simulink model "sampleModel1530"  (R2023a)
settings: Solver=VariableStepAuto  StartTime=0.0  StopTime=10.0  RelTol=1e-3
libraries: hdlsllib x6, simulink x1
settings Model: Creator=user1  LastModifiedBy=user1

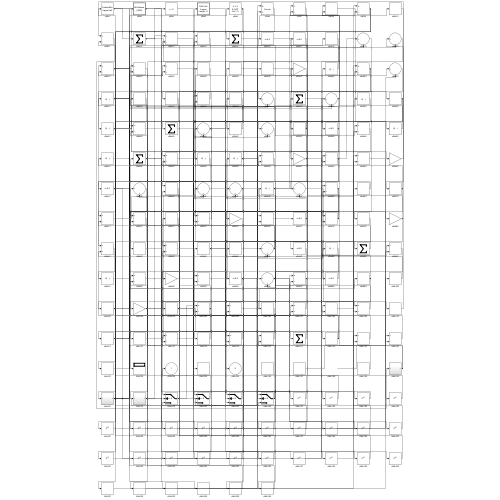
[thumbnail: Simulink's stored preview of the top-level diagram]
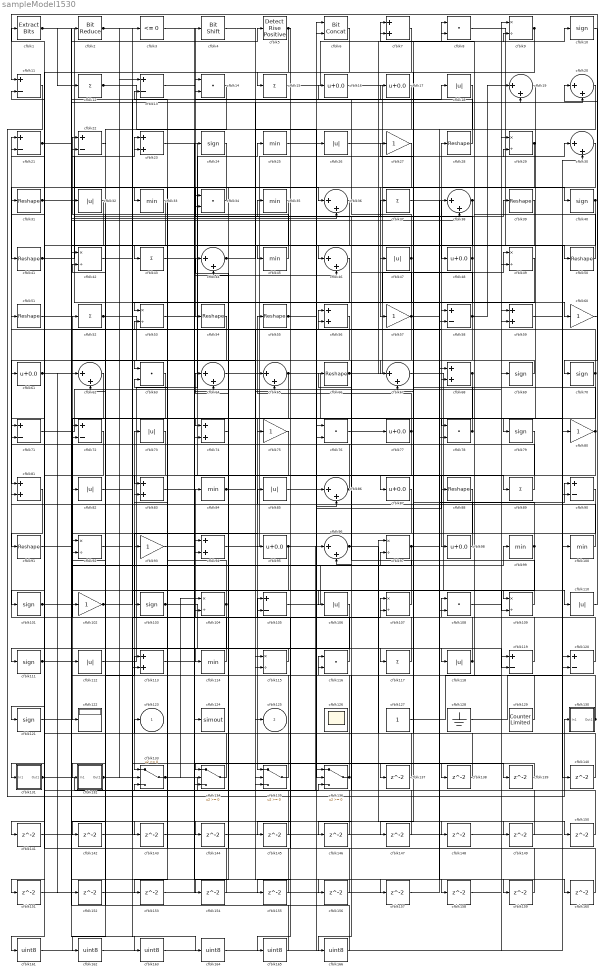
== system sampleModel1530 ==
  cfblk1 : simulink/Logic and Bit Operations/Extract Bits  bitsToExtract=Upper half  numBits=8  bitIdxRange=[0 7]  outScalingMode=Preserve fixed-point scaling
      settings: LibrarySourceBlock=|
      | hdlsllib/Logic and Bit
      | Operations/Extract Bits
  cfblk{10,24,40,69..70,79,101,103,111,121} (10 alike) : Signum
  cfblk{25,33,35,45,84,99..100,114} (8 alike) : MinMax
  cfblk{27,57,60,75,80,93,102} (7 alike) : Gain
  cfblk{9,29,42,49,53,92,97,104,107,109,115} (11 alike) : Product  Inputs=*/  RndMeth=Zero  SaturateOnIntegerOverflow=on
  cfblk{11,13,21..22,58,71..72,90,105,119..120} (11 alike) : Sum  Inputs=+-
  cfblk{18,26,32,47,73,82,85,106,110,112,118} (11 alike) : Abs  SaturateOnIntegerOverflow=off
  cfblk{8,14,34,63,76,78,108,116} (8 alike) : DotProduct  OutDataTypeStr=Inherit: Inherit via internal rule
  cfblk{7,23,56,59,68,74,81,83,94,113} (10 alike) : Sum
  cfblk{12,15,37,43,52,89,117} (7 alike) : Sum  Inputs=+
  cfblk122 : Display
  cfblk124 : ToWorkspace  VariableName=simout  SaveFormat=Timeseries  SampleTime=-1
  cfblk126 : Scope
      settings: Floating=on
  cfblk127 : Constant  SampleTime=-1
  cfblk128 : Ground
  cfblk129 : hdlsllib/Sources/Counter Limited  uplimit=7  tsamp=-1
  cfblk130 : Subsystem
      settings: LibrarySourceBlock=|
      | hdlsllib/Ports &
      | Subsystems/Subsystem
  cfblk131 : Subsystem
      settings: LibrarySourceBlock=|
      | hdlsllib/Ports &
      | Subsystems/Subsystem
  cfblk132 : Subsystem
      settings: LibrarySourceBlock=|
      | hdlsllib/Ports &
      | Subsystems/Subsystem
  cfblk{133..136} (4 alike) : Switch  SaturateOnIntegerOverflow=off  InputSameDT=off
  cfblk{137..160} (24 alike) : Delay  SampleTime=1
  cfblk{16..17,48,61,77,87,95,98} (8 alike) : Bias  Bias=0.0  SaturateOnIntegerOverflow=off
  cfblk{161..166} (6 alike) : DataTypeConversion  OutDataTypeStr=uint8  SaturateOnIntegerOverflow=off  RndMeth=Floor
  cfblk{19..20,30,36,38,44,46,62,64..65,67,86,96} (13 alike) : Sum  Inputs=|++
  cfblk2 : hdlsllib/Logic and Bit Operations/Bit Reduce  mode=AND
  cfblk{28,31,39,41,50..51,54..55,66,88,91} (11 alike) : Reshape
  cfblk3 : hdlsllib/Logic and Bit Operations/Compare To Zero  relop=<=  OutDataTypeStr=boolean
  cfblk4 : hdlsllib/Logic and Bit Operations/Bit Shift  mode=Shift Left Logical  N=0
  cfblk5 : hdlsllib/Logic and Bit Operations/Detect Rise Positive  vinit=0  OutDataTypeStr=boolean
  cfblk6 : hdlsllib/Logic and Bit Operations/Bit Concat  numInputs=2
  cfblk123 : Outport  VectorParamsAs1DForOutWhenUnconnected=off
  cfblk125 : Outport  Port=2  VectorParamsAs1DForOutWhenUnconnected=off
  wires:
  cfblk70/1 -> cfblk135/1, cfblk31/1
  cfblk115/1 -> cfblk114/1
  cfblk130/1(Out1) -> cfblk116/1, cfblk8/2
  cfblk66/1 -> cfblk49/1, cfblk9/2, cfblk166/1
  cfblk48/1 -> cfblk4/1, cfblk113/2
  cfblk67/1 -> cfblk110/1
  cfblk34/1 -> cfblk33/1
  cfblk94/1 -> cfblk30/1
  cfblk131/1(Out1) -> cfblk96/1, cfblk23/2, cfblk99/1, cfblk113/1, cfblk156/1
  cfblk117/1 -> cfblk52/1
  cfblk76/1 -> cfblk77/1
  cfblk63/1 -> cfblk122/1
  cfblk101/1 -> cfblk38/2, cfblk143/1
  cfblk106/1 -> cfblk111/1
  cfblk120/1 -> cfblk84/1
  cfblk19/1 -> cfblk79/1
  cfblk62/1 -> cfblk82/1
  cfblk90/1 -> cfblk133/1
  cfblk23/1 -> cfblk98/1
  cfblk60/1 -> cfblk11/1
  cfblk2/1 -> cfblk109/2, cfblk137/1
  cfblk99/1 -> cfblk102/1, cfblk27/1
  cfblk69/1 -> cfblk63/1
  cfblk17/1 -> cfblk135/2
  cfblk89/1 -> cfblk62/1
  cfblk112/1 -> cfblk25/1
  cfblk109/1 -> cfblk35/1
  cfblk80/1 -> cfblk28/1, cfblk145/1
  cfblk24/1 -> cfblk54/1
  cfblk118/1 -> cfblk108/1, cfblk51/1
  cfblk68/1 -> cfblk132/1(In1), cfblk134/3
  cfblk41/1 -> cfblk23/1, cfblk39/1, cfblk124/1
  cfblk74/1 -> cfblk44/1
  cfblk1/1 -> cfblk60/1, cfblk12/1, cfblk78/1
  cfblk114/1 -> cfblk73/1
  cfblk35/1 -> cfblk112/1
  cfblk119/1 -> cfblk21/1
  cfblk133/1 -> cfblk136/3, cfblk104/1
  cfblk29/1 -> cfblk57/1, cfblk41/1
  cfblk51/1 -> cfblk95/1
  cfblk71/1 -> cfblk49/2
  cfblk7/1 -> cfblk121/1
  cfblk15/1 -> cfblk10/1
  cfblk81/1 -> cfblk91/1
  cfblk54/1 -> cfblk81/1
  cfblk108/1 -> cfblk59/1
  cfblk39/1 -> cfblk46/1
  cfblk47/1 -> cfblk14/1, cfblk43/1, cfblk165/1
  cfblk95/1 -> cfblk26/1, cfblk104/2, cfblk88/1
  cfblk5/1 -> cfblk15/1, cfblk155/1
  cfblk38/1 -> cfblk8/1, cfblk94/2
  cfblk45/1 -> cfblk22/1
  cfblk83/1 -> cfblk46/2
  cfblk53/1 -> cfblk76/2
  cfblk50/1 -> cfblk7/1
  cfblk96/1 -> cfblk66/1, cfblk148/1, cfblk149/1
  cfblk27/1 -> cfblk44/2
  cfblk86/1 -> cfblk32/1, cfblk71/2
  cfblk37/1 -> cfblk48/1
  cfblk21/1 -> cfblk2/1, cfblk65/2, cfblk14/2, cfblk64/2
  cfblk30/1 -> cfblk83/1
  cfblk127/1 -> cfblk59/2
  cfblk98/1 -> cfblk68/2
  cfblk132/1(Out1) -> cfblk107/1, cfblk3/1, cfblk158/1
  cfblk64/1 -> cfblk55/1
  cfblk46/1 -> cfblk53/1
  cfblk11/1 -> cfblk130/1(In1)
  cfblk103/1 -> cfblk24/1, cfblk118/1
  cfblk44/1 -> cfblk115/1, cfblk19/2
  cfblk113/1 -> cfblk107/2
  cfblk110/1 -> cfblk20/1
  cfblk111/1 -> cfblk20/2, cfblk56/2, cfblk5/1
  cfblk77/1 -> cfblk103/1, cfblk65/1
  cfblk78/1 -> cfblk7/2, cfblk74/1
  cfblk128/1 -> cfblk100/1
  cfblk49/1 -> cfblk67/1
  cfblk121/1 -> cfblk22/2
  cfblk129/1 -> cfblk63/2
  cfblk88/1 -> cfblk96/2
  cfblk135/1 -> cfblk62/2
  cfblk10/1 -> cfblk70/1
  cfblk9/1 -> cfblk61/1, cfblk72/2, cfblk87/1
  cfblk8/1 -> cfblk80/1
  cfblk136/1 -> cfblk134/1, cfblk92/1
  cfblk18/1 -> cfblk45/1
  cfblk107/1 -> cfblk85/1
  cfblk12/1 -> cfblk86/1, cfblk13/1
  cfblk104/1 -> cfblk131/1(In1), cfblk13/2
  cfblk13/1 -> cfblk134/2
  cfblk79/1 -> cfblk135/3
  cfblk134/1 -> cfblk123/1
  cfblk52/1 -> cfblk125/1, cfblk18/1
  cfblk100/1 -> cfblk81/2
  cfblk55/1 -> cfblk86/2, cfblk29/2
  cfblk65/1 -> cfblk93/1, cfblk120/2
  cfblk105/1 -> cfblk97/2
  cfblk85/1 -> cfblk58/1
  cfblk22/1 -> cfblk72/1
  cfblk26/1 -> cfblk58/2
  cfblk116/1 -> cfblk105/1
  cfblk84/1 -> cfblk56/1, cfblk109/1
  cfblk16/1 -> cfblk40/1
  cfblk97/1 -> cfblk90/1, cfblk92/2
  cfblk28/1 -> cfblk16/1
  cfblk57/1 -> cfblk115/2, cfblk34/2, cfblk160/1
  cfblk92/1 -> cfblk119/2
  cfblk56/1 -> cfblk71/1
  cfblk87/1 -> cfblk106/1
  cfblk43/1 -> cfblk89/1
  cfblk20/1 -> cfblk108/2
  cfblk33/1 -> cfblk101/1
  cfblk58/1 -> cfblk17/1, cfblk19/1, cfblk146/1, cfblk147/1
  cfblk61/1 -> cfblk78/2, cfblk150/1, cfblk152/1
  cfblk40/1 -> cfblk47/1, cfblk74/2
  cfblk102/1 -> cfblk117/1, cfblk37/1
  cfblk31/1 -> cfblk75/1, cfblk50/1, cfblk36/1, cfblk36/2
  cfblk137/1 -> cfblk97/1
  cfblk25/1 -> cfblk138/1
  cfblk138/1 -> cfblk11/2
  cfblk93/1 -> cfblk139/1
  cfblk139/1 -> cfblk136/2
  cfblk59/1 -> cfblk140/1
  cfblk140/1 -> cfblk67/2
  cfblk32/1 -> cfblk141/1
  cfblk141/1 -> cfblk90/2
  cfblk73/1 -> cfblk142/1
  cfblk142/1 -> cfblk133/2
  cfblk143/1 -> cfblk136/1
  cfblk82/1 -> cfblk144/1
  cfblk144/1 -> cfblk119/1
  cfblk145/1 -> cfblk1/1
  cfblk146/1 -> cfblk34/1
  cfblk147/1 -> cfblk53/2
  cfblk148/1 -> cfblk30/2
  cfblk149/1 -> cfblk116/2
  cfblk150/1 -> cfblk9/1
  cfblk72/1 -> cfblk151/1
  cfblk151/1 -> cfblk76/1
  cfblk152/1 -> cfblk38/1
  cfblk75/1 -> cfblk153/1
  cfblk153/1 -> cfblk94/1
  cfblk36/1 -> cfblk154/1
  cfblk154/1 -> cfblk21/2
  cfblk155/1 -> cfblk133/3
  cfblk156/1 -> cfblk105/2
  cfblk3/1 -> cfblk157/1
  cfblk157/1 -> cfblk68/1
  cfblk158/1 -> cfblk29/1
  cfblk4/1 -> cfblk159/1
  cfblk159/1 -> cfblk83/2
  cfblk160/1 -> cfblk64/1
  cfblk6/1 -> cfblk161/1
  cfblk161/1 -> cfblk120/1
  cfblk14/1 -> cfblk162/1
  cfblk162/1 -> cfblk6/1
  cfblk91/1 -> cfblk163/1
  cfblk163/1 -> cfblk6/2
  cfblk42/1 -> cfblk164/1
  cfblk164/1 -> cfblk69/1
  cfblk165/1 -> cfblk42/1
  cfblk166/1 -> cfblk42/2

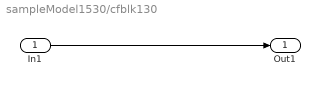
== system sampleModel1530/cfblk130 ==
  In1 : Inport
  Out1 : Outport
  wires:
  In1/1 -> Out1/1

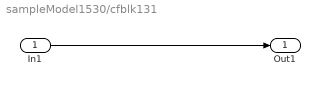
== system sampleModel1530/cfblk131 ==
  In1 : Inport
  Out1 : Outport
  wires:
  In1/1 -> Out1/1

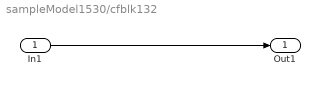
== system sampleModel1530/cfblk132 ==
  In1 : Inport
  Out1 : Outport
  wires:
  In1/1 -> Out1/1
